simulink model "alimentacion"  (R2023b)
settings: Solver=VariableStepAuto  StartTime=0.0  StopTime=15.0  RelTol=1e-3
libraries: simulink x1
settings Model: Creator=Matlab  LastModifiedBy=erwinplanck
settings ModelReferenceCC: EnableRefExpFcnMdlSchedulingChecks=on

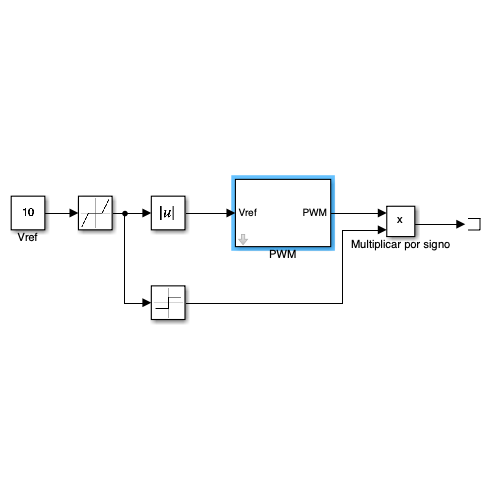
[thumbnail: Simulink's stored preview of the top-level diagram]
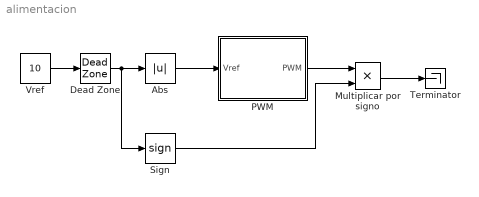
== system alimentacion ==
  Abs : Abs  SaturateOnIntegerOverflow=off
  Dead Zone : DeadZone
  Multiplicar por signo : Product
  PWM : Subsystem  mask{T=0.001, Vmax=12}
      mask prompts: T "Periodo"; Vmax "Voltaje"
  Sign : Signum
  Terminator : Terminator
  Vref : Constant  Value=10
  wires:
  Sign/1 -> Multiplicar por signo/2
  PWM/1(PWM) -> Multiplicar por signo/1
  Multiplicar por signo/1 -> Terminator/1
  Abs/1 -> PWM/1(Vref)
  Vref/1 -> Dead Zone/1
  Dead Zone/1 -> Sign/1, Abs/1

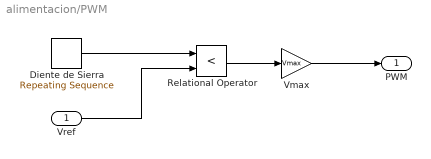
== system alimentacion/PWM ==
  Vref : Inport
  "Diente de Sierra " : simulink/Sources/Repeating Sequence  rep_seq_t=linspace(0, T, 100)  rep_seq_y=linspace(0,Vmax,100)
  Relational Operator : RelationalOperator  Operator=<  OutDataTypeStr=boolean  RndMeth=Simplest  InputSameDT=off
  Vmax : Gain  Gain=Vmax
  PWM : Outport
  wires:
  Vmax/1 -> PWM/1
  Vref/1 -> Relational Operator/2
  "Diente de Sierra "/1 -> Relational Operator/1
  Relational Operator/1 -> Vmax/1
